simulink model "Transl_id"  (R2017b)
settings: Solver=VariableStepAuto  StartTime=0.0  StopTime=inf  FixedStep=10e-3  RelTol=1e-3
values from neighbouring files (symbols this model uses):
  imu = rossubscriber('/imu')    [identification.m]
undefined symbols (not defined in the file or in its folder): Angular, Linear
libraries: robotlib x3, simulink x2, commseqgen3 x1
settings Model: Creator=alic  LastModifiedBy=alic

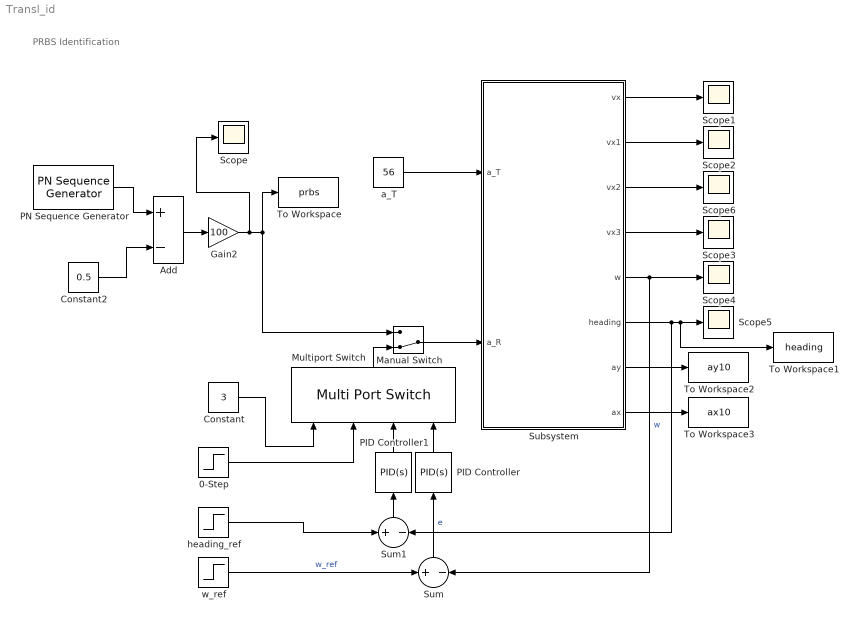
== system Transl_id ==
  note: PRBS Identification
  0-Step : Step  Time=0  After=0  SampleTime=0
  Add : Sum  Inputs=+-
  Constant : Constant  Value=3
  Constant2 : Constant  Value=0.5
  Gain2 : Gain  Gain=100
  Manual Switch : ManualSwitch  CurrentSetting=0
  Multiport Switch : MultiPortSwitch
  PID Controller : simulink/Continuous/PID Controller  Controller=PID  TimeDomain=Continuous-time  SampleTime=-1  IntegratorMethod=Forward Euler  FilterMethod=Forward Euler  Form=Parallel  UseFilter=on  ControllerParametersSource=internal  P=0.3  I=0  D=0  N=100  InitialConditionSource=internal  InitialConditionForIntegrator=0  InitialConditionForFilter=0  ExternalReset=none  LimitOutput=off  UpperSaturationLimit=inf  LowerSaturationLimit=-inf  LinearizeAsGain=on  AntiWindupMode=none  Kb=1  TrackingMode=off  Kt=1  PParamMin=[]  PParamMax=[]  IParamMin=[]  IParamMax=[]  DParamMin=[]  DParamMax=[]  NParamMin=[]  NParamMax=[]  KbParamMin=[]  KbParamMax=[]  KtParamMin=[]  KtParamMax=[]  POutMin=[]  POutMax=[]  IOutMin=[]  IOutMax=[]  DOutMin=[]  DOutMax=[]  NOutMin=[]  NOutMax=[]  KbOutMin=[]  KbOutMax=[]  KtOutMin=[]  KtOutMax=[]  IntegratorOutMin=[]  IntegratorOutMax=[]  FilterOutMin=[]  FilterOutMax=[]  SumOutMin=[]  SumOutMax=[]  SumI1OutMin=[]  SumI1OutMax=[]  SumI2OutMin=[]  SumI2OutMax=[]  SumI3OutMin=[]  SumI3OutMax=[]  SumDOutMin=[]  SumDOutMax=[]  SaturationOutMin=[]  SaturationOutMax=[]  IntegratorContinuousStateAttributes=''  IntegratorStateMustResolveToSignalObject=off  IntegratorRTWStateStorageClass=Auto  FilterContinuousStateAttributes=''  FilterStateMustResolveToSignalObject=off  FilterRTWStateStorageClass=Auto  DifferentiatorICPrevScaledInput=0  DifferentiatorOutMin=[]  DifferentiatorOutMax=[]  InitialConditionSetting=State (most efficient)  FilterDiffOutCoefMin=[]  FilterDiffOutCoefMax=[]  SumDenOutMin=[]  SumDenOutMax=[]  SumNumOutMin=[]  SumNumOutMax=[]  ReciprocalOutMin=[]  ReciprocalOutMax=[]  DivideOutMin=[]  DivideOutMax=[]  TunerSelectOption=Transfer Function Based (PID Tuner App)
  PID Controller1 : simulink/Continuous/PID Controller  Controller=PID  TimeDomain=Continuous-time  SampleTime=-1  IntegratorMethod=Forward Euler  FilterMethod=Forward Euler  Form=Ideal  UseFilter=on  ControllerParametersSource=internal  P=0.2  I=4  D=1  N=100  InitialConditionSource=internal  InitialConditionForIntegrator=0  InitialConditionForFilter=0  ExternalReset=none  LimitOutput=off  UpperSaturationLimit=inf  LowerSaturationLimit=-inf  LinearizeAsGain=on  AntiWindupMode=none  Kb=1  TrackingMode=off  Kt=1  PParamMin=[]  PParamMax=[]  IParamMin=[]  IParamMax=[]  DParamMin=[]  DParamMax=[]  NParamMin=[]  NParamMax=[]  KbParamMin=[]  KbParamMax=[]  KtParamMin=[]  KtParamMax=[]  POutMin=[]  POutMax=[]  IOutMin=[]  IOutMax=[]  DOutMin=[]  DOutMax=[]  NOutMin=[]  NOutMax=[]  KbOutMin=[]  KbOutMax=[]  KtOutMin=[]  KtOutMax=[]  IntegratorOutMin=[]  IntegratorOutMax=[]  FilterOutMin=[]  FilterOutMax=[]  SumOutMin=[]  SumOutMax=[]  SumI1OutMin=[]  SumI1OutMax=[]  SumI2OutMin=[]  SumI2OutMax=[]  SumI3OutMin=[]  SumI3OutMax=[]  SumDOutMin=[]  SumDOutMax=[]  SaturationOutMin=[]  SaturationOutMax=[]  IntegratorContinuousStateAttributes=''  IntegratorStateMustResolveToSignalObject=off  IntegratorRTWStateStorageClass=Auto  FilterContinuousStateAttributes=''  FilterStateMustResolveToSignalObject=off  FilterRTWStateStorageClass=Auto  DifferentiatorICPrevScaledInput=0  DifferentiatorOutMin=[]  DifferentiatorOutMax=[]  InitialConditionSetting=State (most efficient)  FilterDiffOutCoefMin=[]  FilterDiffOutCoefMax=[]  SumDenOutMin=[]  SumDenOutMax=[]  SumNumOutMin=[]  SumNumOutMax=[]  ReciprocalOutMin=[]  ReciprocalOutMax=[]  DivideOutMin=[]  DivideOutMax=[]  TunerSelectOption=Transfer Function Based (PID Tuner App)
  PN Sequence Generator : commseqgen3/PN Sequence Generator  poly='z^8 + z^6 + z^5 + z^4 + 1'  ini_sta=[0 0 0 0 0 0 0 1]  outBitMaskSource=Dialog parameter  shift=0  outVarSiz=off  maxOutSizeMode=Dialog parameter  maxOutSize=[10 1]  Ts=-1  sampPerFrame=1  reset=off  bitPackedOutputs=off  outDataType=double  numPackedBits=8  bitPackDataSigned=off  bitPackedOutDType=double
      settings: SourceProductName=Communications System Toolbox
  Scope{,1..6} (7 alike) : Scope
  Subsystem : Subsystem
  Sum : Sum  Inputs=+-
  Sum1 : Sum  Inputs=+-
  To Workspace : ToWorkspace  VariableName=prbs  SaveFormat=Timeseries  SampleTime=-1
  To Workspace1 : ToWorkspace  VariableName=heading  SaveFormat=Timeseries  SampleTime=-1
  To Workspace2 : ToWorkspace  VariableName=ay10  SaveFormat=Timeseries  SampleTime=-1
  To Workspace3 : ToWorkspace  VariableName=ax10  SaveFormat=Timeseries  SampleTime=-1
  a_T : Constant  Value=56
  heading_ref : Step  Time=0  After=0  SampleTime=0
  w_ref : Step  Time=0  After=0.1  SampleTime=0
  wires:
  Subsystem/1(vx) -> Scope1/1
  Subsystem/2(vx1) -> Scope2/1
  Subsystem/3(vx2) -> Scope6/1
  Subsystem/4(vx3) -> Scope3/1
  Subsystem/5(w) -> Sum/2, Scope4/1  "w"
  w_ref/1 -> Sum/1  "w_ref"
  heading_ref/1 -> Sum1/1
  Sum1/1 -> PID Controller1/1
  Sum/1 -> PID Controller/1  "e"
  PID Controller/1 -> Multiport Switch/4
  PID Controller1/1 -> Multiport Switch/3
  Constant/1 -> Multiport Switch/1
  0-Step/1 -> Multiport Switch/2
  Multiport Switch/1 -> Manual Switch/2
  Constant2/1 -> Add/2
  PN Sequence Generator/1 -> Add/1
  Add/1 -> Gain2/1
  Gain2/1 -> Scope/1, Manual Switch/1, To Workspace/1
  Subsystem/7(ay) -> To Workspace2/1
  Subsystem/8(ax) -> To Workspace3/1
  Subsystem/6(heading) -> To Workspace1/1, Scope5/1, Sum1/2
  Manual Switch/1 -> Subsystem/2(a_R)
  a_T/1 -> Subsystem/1(a_T)

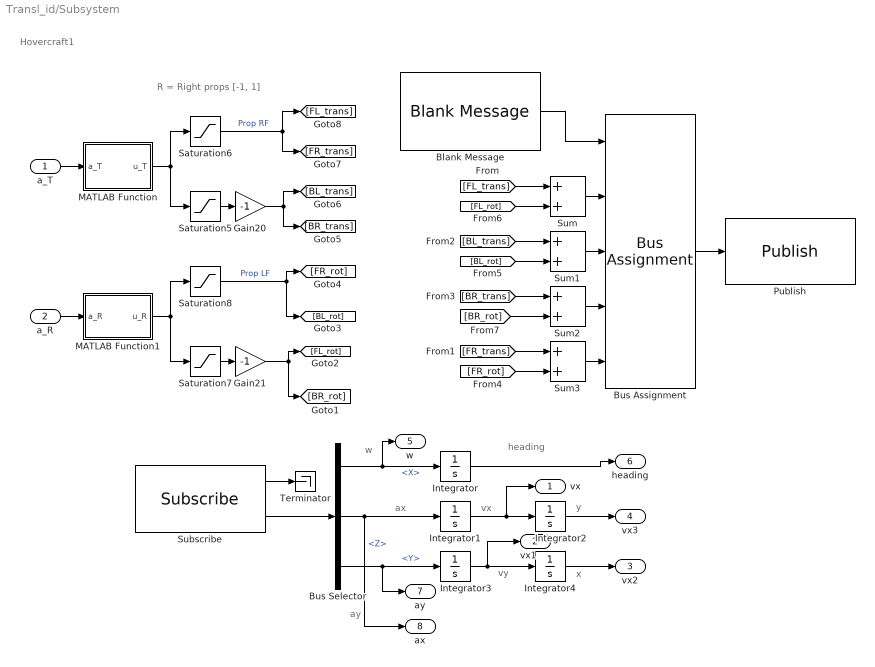
== system Transl_id/Subsystem ==
  note: Hovercraft1
  note: y
  note: x
  note: vy
  note: ay
  note: R = Right props [-1, 1]
  note: w
  note: heading
  note: ax
  note: vx
  a_T : Inport
  a_R : Inport  Port=2
  Blank Message : robotlib/Blank Message  SourceLibraryInfo=This block requires Robotics System Toolbox  messageType=geometry_msgs/Twist  SampleTime=inf
      settings: SourceProductBaseCode=RO
  Bus Assignment : BusAssignment  AssignedSignals=Linear.X,Linear.Y,Angular.X,Angular.Y
  Bus Selector : BusSelector  OutputSignals=AngularVelocity.X,LinearAcceleration.Z,LinearAcceleration.Y
  Gain20 : Gain  Gain=-1
  Gain21 : Gain  Gain=-1
  Integrator{,1..4} (5 alike) : Integrator
  MATLAB Function : MATLAB Function  TreatAsAtomicUnit=on
  MATLAB Function1 : MATLAB Function  TreatAsAtomicUnit=on
  Publish : robotlib/Publish  SourceLibraryInfo=This block requires Robotics System Toolbox  topicSource=Select from ROS network  topic=/cmd_vel  messageType=geometry_msgs/Twist  messageQueueLength=1
      settings: SourceProductBaseCode=RO
  Saturation5 : Saturate  UpperLimit=0  LowerLimit=-100
  Saturation6 : Saturate  UpperLimit=100  LowerLimit=0
  Saturation7 : Saturate  UpperLimit=0  LowerLimit=-100
  Saturation8 : Saturate  UpperLimit=100  LowerLimit=0
  Subscribe : robotlib/Subscribe  SourceLibraryInfo=This block requires Robotics System Toolbox  topicSource=Select from ROS network  topic=/imu  messageType=sensor_msgs/Imu  sampleTime=-1  messageQueueLength=1
      settings: SourceProductBaseCode=RO
  Sum{,1..3} (4 alike) : Sum
  Terminator : Terminator
  vx : Outport
  vx1 : Outport  Port=2
  vx2 : Outport  Port=3
  vx3 : Outport  Port=4
  w : Outport  Port=5
  heading : Outport  Port=6
  ay : Outport  Port=7
  ax : Outport  Port=8
  wires:
  Integrator/1 -> heading/1
  Integrator4/1 -> vx2/1
  Integrator3/1 -> vx1/1, Integrator4/1
  Saturation7/1 -> Gain21/1
  Bus Assignment/1 -> Publish/1
  Subscribe/1 -> Terminator/1
  Subscribe/2 -> Bus Selector/1
  Integrator2/1 -> vx3/1
  Integrator1/1 -> vx/1, Integrator2/1
  Bus Selector/1 -> Integrator/1, w/1  "<X>"
  Blank Message/1 -> Bus Assignment/1
  Saturation5/1 -> Gain20/1
  Bus Selector/2 -> Integrator1/1, ax/1  "<Z>"
  Bus Selector/3 -> Integrator3/1, ay/1  "<Y>"
  Gain21/1 -> [FL_rot], [BR_rot]
  Saturation8/1 -> [BL_rot], [FR_rot]  "Prop LF"
  Gain20/1 -> [BR_trans], [BL_trans]
  Saturation6/1 -> [FR_trans], [FL_trans]  "Prop RF"
  [FL_rot] -> Sum/2
  Sum/1 -> Bus Assignment/2
  Sum1/1 -> Bus Assignment/3
  Sum2/1 -> Bus Assignment/4
  Sum3/1 -> Bus Assignment/5
  [FL_trans] -> Sum/1
  [FR_trans] -> Sum3/1
  [FR_rot] -> Sum3/2
  [BL_rot] -> Sum1/2
  [BL_trans] -> Sum1/1
  [BR_trans] -> Sum2/1
  [BR_rot] -> Sum2/2
  a_T/1 -> MATLAB Function/1(a_T)
  MATLAB Function/1(u_T) -> Saturation6/1, Saturation5/1
  a_R/1 -> MATLAB Function1/1(a_R)
  MATLAB Function1/1(u_R) -> Saturation7/1, Saturation8/1

== matlab function Transl_id/Subsystem/MATLAB Function1 ==
  data: a_R input; u_R output
function u_R = inv_map_R(a_R)

== matlab function Transl_id/Subsystem/MATLAB Function ==
  data: a_T input; u_T output
function u_T = inv_map_T(a_T)
